simulink model "SineWave"  (R2019b)
settings: Solver=VariableStepAuto  StartTime=0.0  StopTime=10.0  MaxStep=0.01  RelTol=1e-3
settings Model: Creator=Kudi Okerulu  LastModifiedBy=Kudi Okerulu
settings SFSimCC: CustomCodeUndefinedFunction=UseInterfaceOnly

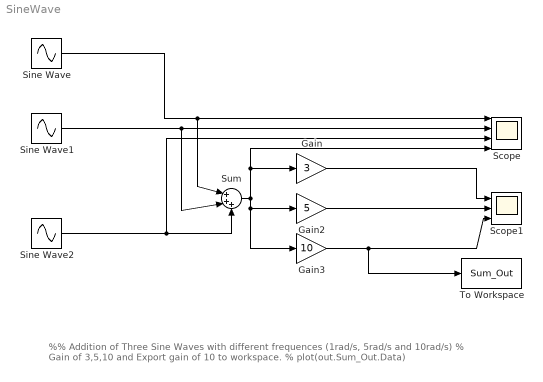
== system SineWave ==
  note: %% Addition of Three Sine Waves with different frequences (1rad/s, 5rad/s and 10rad/s)
      | %    Gain of 3,5,10 and Export gain of 10 to workspace.
      | %    plot(out.Sum_Out.Data)
  Gain : Gain  Gain=3
  Gain2 : Gain  Gain=5
  Gain3 : Gain  Gain=10
  Scope : Scope  NumInputPorts=4
  Scope1 : Scope  NumInputPorts=3
  Sine Wave : Sin  SampleTime=0
  Sine Wave1 : Sin  Frequency=5  SampleTime=0
  Sine Wave2 : Sin  Frequency=10  SampleTime=0
  Sum : Sum  Inputs=|+++
  To Workspace : ToWorkspace  VariableName=Sum_Out  SaveFormat=Timeseries  SampleTime=-1
  wires:
  Sine Wave/1 -> Sum/1, Scope/1
  Sine Wave1/1 -> Sum/2, Scope/2
  Sine Wave2/1 -> Sum/3, Scope/3
  Sum/1 -> Gain2/1, Gain3/1, Gain/1, Scope/4
  Gain/1 -> Scope1/1
  Gain2/1 -> Scope1/2
  Gain3/1 -> To Workspace/1, Scope1/3
